simulink model "test"  (R2020a)
settings: Solver=VariableStepAuto  StartTime=0.0  StopTime=10  FixedStep=0.001  RelTol=1e-3
values from neighbouring files (symbols this model uses):
  den1 = [1 b*(i+m*l^2)/q1 -(M+m)*m*g*l/q1 -b*m*g*l/q1]    [parameter.m]
  num1 = [m*l/q1 0]    [parameter.m]
libraries: simulink x3, rllib x1
settings Model: Creator=Preload  LastModifiedBy=User
settings DataIOCC: ReturnWorkspaceOutputs=off
settings DebuggingCC: ArithmeticOperatorsInVariantConditions=warning
settings SFSimCC: SimUseLocalCustomCode=off  CustomCodeUndefinedFunction=UseInterfaceOnly
settings RTWCC: RTWUseLocalCustomCode=off

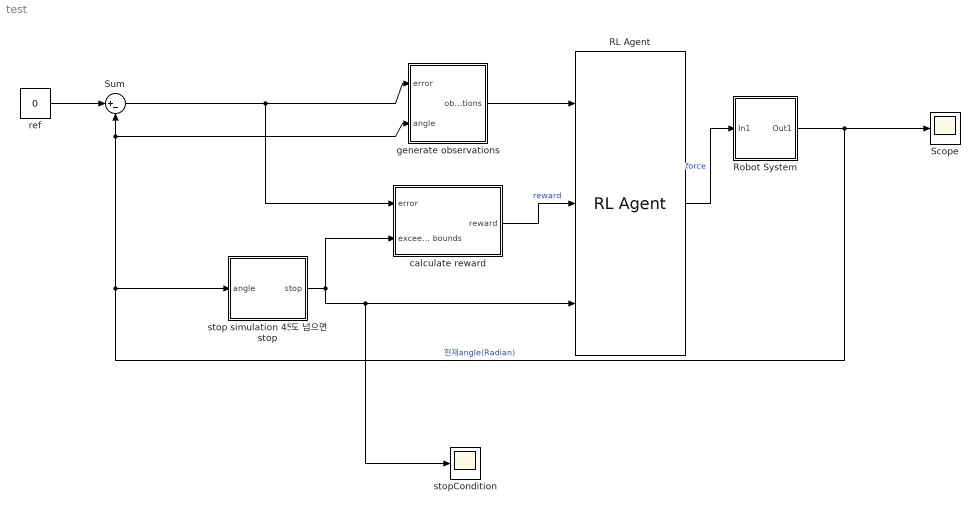
== system test ==
  RL Agent : rllib/RL Agent  Agent=agent  ProvideReward=on  ProvideIsDone=on  ProvideCumRwd=off  TreatAsDirectFeedthrough=on  CollectLoggedSignals=on  CollectModelStates=on
  Robot System : Subsystem
  Scope : Scope
  Sum : Sum  Inputs=|+-
  calculate reward : Subsystem
  generate observations : Subsystem
  ref : Constant  Value=0
  stop simulation 45도 넘으면 stop : Subsystem
  stopCondition : Scope
  wires:
  ref/1 -> Sum/1
  RL Agent/1 -> Robot System/1(In1)  "force"
  stop simulation 45도 넘으면 stop/1(stop) -> stopCondition/1, RL Agent/3, calculate reward/2(exceeds bounds)
  Sum/1 -> calculate reward/1(error), generate observations/1(error)
  Robot System/1(Out1) -> Scope/1, stop simulation 45도 넘으면 stop/1(angle), Sum/2, generate observations/2(angle)  "현재angle(Radian)"
  generate observations/1(observations) -> RL Agent/1
  calculate reward/1(reward) -> RL Agent/2  "reward"

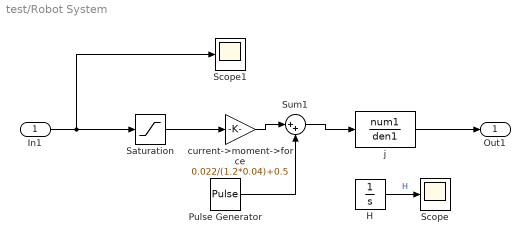
== system test/Robot System ==
  In1 : Inport
  H : Integrator  LimitOutput=on  LowerSaturationLimit=0
  Pulse Generator : DiscretePulseGenerator  PulseType=Time based  Period=10  PulseWidth=0.1  PhaseDelay=0.1
  Saturation : Saturate  UpperLimit=12  LowerLimit=-12
  Scope : Scope
  Scope1 : Scope
  Sum1 : Sum  Inputs=|++
  current->moment->force : Gain  Gain=0.022/(1.2*0.04)+0.5
  j : TransferFcn  Numerator=num1  Denominator=den1
  Out1 : Outport
  wires:
  In1/1 -> Saturation/1, Scope1/1
  j/1 -> Out1/1
  H/1 -> Scope/1  "H"
  Saturation/1 -> current->moment->force/1
  Pulse Generator/1 -> Sum1/2
  current->moment->force/1 -> Sum1/1
  Sum1/1 -> j/1

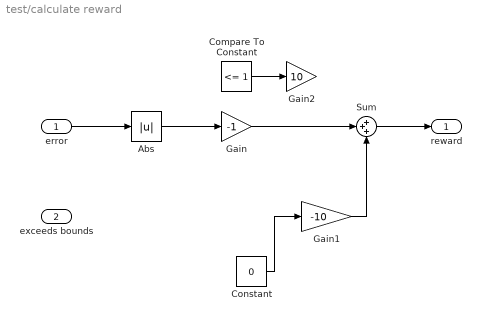
== system test/calculate reward ==
  error : Inport
  exceeds bounds : Inport  Port=2
  Abs : Abs
  Compare To Constant : simulink/Logic and Bit Operations/Compare To Constant  relop=<=  const=1  OutDataTypeStr=boolean
  Constant : Constant  Value=0
  Gain : Gain  Gain=-1
  Gain1 : Gain  Gain=-10
  Gain2 : Gain  Gain=10
  Sum : Sum  Inputs=+++
  reward : Outport  VectorParamsAs1DForOutWhenUnconnected=off
  wires:
  error/1 -> Abs/1
  Abs/1 -> Gain/1
  Sum/1 -> reward/1
  Compare To Constant/1 -> Gain2/1
  Gain/1 -> Sum/2
  Gain1/1 -> Sum/3
  Constant/1 -> Gain1/1

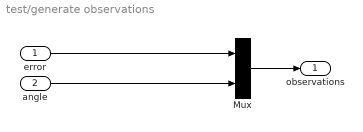
== system test/generate observations ==
  error : Inport
  angle : Inport  Port=2
  Mux : Mux  Inputs=2
  observations : Outport  VectorParamsAs1DForOutWhenUnconnected=off
  wires:
  error/1 -> Mux/1
  angle/1 -> Mux/2
  Mux/1 -> observations/1

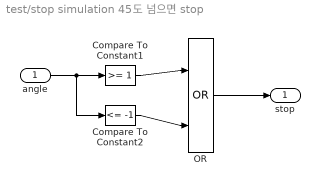
== system test/stop simulation 45도 넘으면 stop ==
  angle : Inport
  Compare To Constant1 : simulink/Logic and Bit Operations/Compare To Constant  relop=>=  const=1  OutDataTypeStr=boolean
  Compare To Constant2 : simulink/Logic and Bit Operations/Compare To Constant  relop=<=  const=-1  OutDataTypeStr=boolean
  OR : Logic  Operator=OR  IconShape=distinctive  AllPortsSameDT=off  OutDataTypeStr=boolean
  stop : Outport  VectorParamsAs1DForOutWhenUnconnected=off
  wires:
  Compare To Constant2/1 -> OR/2
  angle/1 -> Compare To Constant2/1, Compare To Constant1/1
  OR/1 -> stop/1
  Compare To Constant1/1 -> OR/1
